simulink model "transfer_function_as_block"  (R2023a)
settings: Solver=VariableStepAuto  StartTime=0.0  StopTime=10.0  RelTol=1e-3
undefined symbols (not defined in the file or in its folder): G_D_sim, G_S_sim
libraries: cstblocks x2
settings Model: Creator=pascalbock  LastModifiedBy=pascalbock

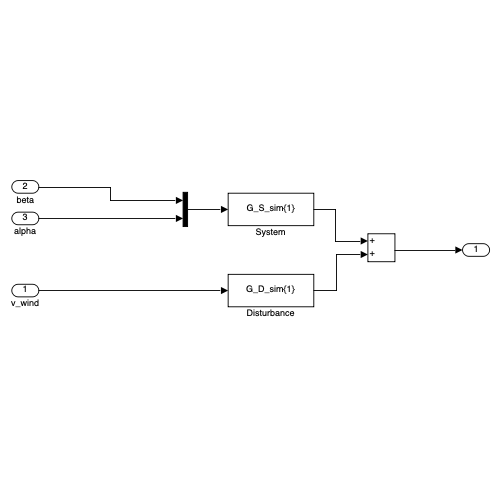
[thumbnail: Simulink's stored preview of the top-level diagram]
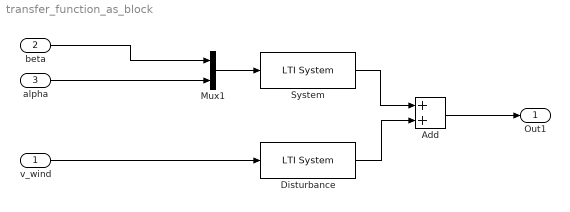
== system transfer_function_as_block ==
  v_wind : Inport
  beta : Inport  Port=2
  alpha : Inport  Port=3
  Add : Sum
  Disturbance : cstblocks/LTI System  sys=G_D_sim{1}  IC=[]
  Mux1 : Mux  Inputs=2
  System : cstblocks/LTI System  sys=G_S_sim{1}  IC=[]
  Out1 : Outport
  wires:
  System/1 -> Add/1
  Add/1 -> Out1/1
  beta/1 -> Mux1/1
  v_wind/1 -> Disturbance/1
  alpha/1 -> Mux1/2
  Mux1/1 -> System/1
  Disturbance/1 -> Add/2
